simulink model "OvenSim"  (R2024a)
settings: Solver=FixedStepAuto  StartTime=0  StopTime=60  FixedStep=0.1  RelTol=1e-3
values from neighbouring files (symbols this model uses):
  A_innerwalls = 1.12    [ovenSimConfig.m]
  convection_loss_coefficient = 0.1    [ovenSimConfig.m]
  epsilon_food = 0.9    [ovenSimConfig.m]
  epsilon_innerWalls = 0.6    [ovenSimConfig.m]
  radiation_loss_coefficient = 0.24    [ovenSimConfig.m]
  sigma = 5.67e-8    (= 5.67e-08)    [ovenSimConfig.m]
undefined symbols (not defined in the file or in its folder): a, b
libraries: fl_lib x10, nesl_utility x8, CustomComponents_lib x1
settings Model: Creator=Jonas Zhou  LastModifiedBy=zhouziyao

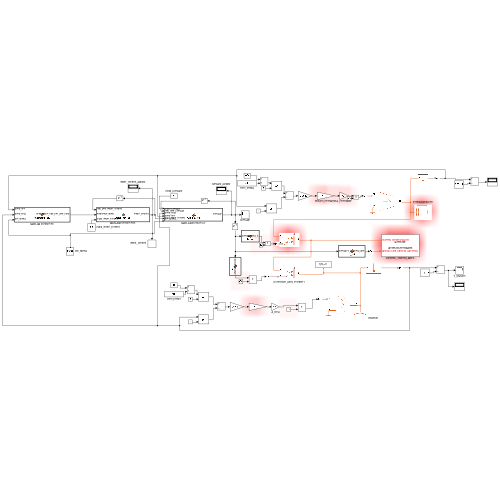
[thumbnail: Simulink's stored preview of the top-level diagram]
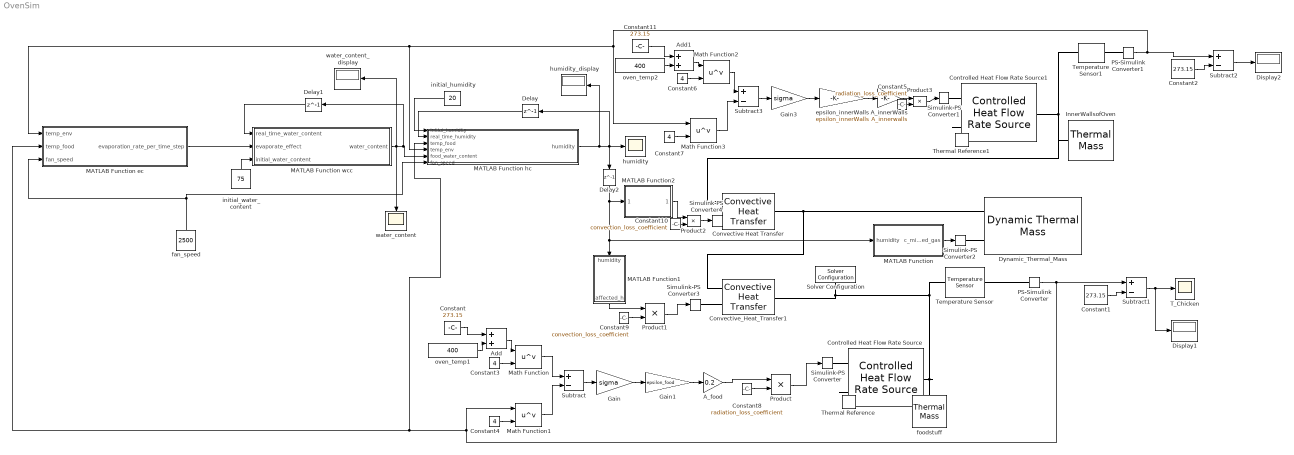
== system OvenSim ==
  A_food : Gain  Gain=0.2
  A_innerWalls : Gain  Gain=A_innerwalls
  Add : Sum
  Add1 : Sum
  Constant{,1..2,11} (4 alike) : Constant  Value=273.15
  Constant10 : Constant  Value=convection_loss_coefficient
  Constant{3..4,6..7} (4 alike) : Constant  Value=4
  Constant5 : Constant  Value=radiation_loss_coefficient
  Constant8 : Constant  Value=radiation_loss_coefficient
  Constant9 : Constant  Value=convection_loss_coefficient
  Controlled Heat Flow Rate Source : fl_lib/Thermal/Thermal Sources/Controlled Heat Flow Rate Source
  Controlled Heat Flow Rate Source1 : fl_lib/Thermal/Thermal Sources/Controlled Heat Flow Rate Source
  Convective Heat Transfer : fl_lib/Thermal/Thermal Elements/Convective Heat Transfer  thermal_type=foundation.enum.constant_variable.variable  area=A_gas m^2  heat_tr_coeff=h_innerwalls W/(K*m^2)  min_heat_tr_coeff=1e-3 W/(K*m^2)  T_specify=off  T_priority=None  T=a-b K  T_nominal_specify=off  T_nominal_value=1  T_nominal_unit=K  Q_specify=off  Q_priority=None  Q=0 W  Q_nominal_specify=off  Q_nominal_value=1  Q_nominal_unit=W
      settings: InternalSimscapePortConfiguration="{\"Bottom\":[],\"Left\":[{\"id\":\"A\",\"label\":\"A\",\"type\":\"foundation.thermal.thermal\"},{\"id\":\"var_heat_tr_coeff\",\"label\":\"K\",\"type\":\"input\"}],\"Right\":[{\"id\":\"B\",\"label\":\"B\",\"type\":\"foundation.thermal.thermal\"}],\"Top\":[]}"
  Convective_Heat_Transfer1 : fl_lib/Thermal/Thermal Elements/Convective Heat Transfer  thermal_type=foundation.enum.constant_variable.variable  area=0.2 m^2  heat_tr_coeff=20 W/(K*m^2)  min_heat_tr_coeff=1e-3 W/(K*m^2)  T_specify=off  T_priority=None  T=a-b K  T_nominal_specify=off  T_nominal_value=1  T_nominal_unit=K  Q_specify=off  Q_priority=None  Q=0 W  Q_nominal_specify=off  Q_nominal_value=1  Q_nominal_unit=W
      settings: InternalSimscapePortConfiguration="{\"Bottom\":[],\"Left\":[{\"id\":\"A\",\"label\":\"A\",\"type\":\"foundation.thermal.thermal\"},{\"id\":\"var_heat_tr_coeff\",\"label\":\"K\",\"type\":\"input\"}],\"Right\":[{\"id\":\"B\",\"label\":\"B\",\"type\":\"foundation.thermal.thermal\"}],\"Top\":[]}"
  Delay : Delay  DelayLength=1  InitialCondition=0
  Delay1 : Delay  DelayLength=1  InitialCondition=0
  Delay2 : Delay  DelayLength=1  InitialCondition=0
  Display1 : Display
  Display2 : Display
  Dynamic_Thermal_Mass : CustomComponents_lib/Dynamic Thermal Mass  mass=m_gas kg  T_specify=on  T_priority=None  T=400 degC  T_nominal_specify=off  T_nominal_value=1  T_nominal_unit=K  Q_specify=off  Q_priority=None  Q=0 W  Q_nominal_specify=off  Q_nominal_value=1  Q_nominal_unit=W
      settings: InternalSimscapePortConfiguration="{\"Bottom\":[],\"Left\":[{\"id\":\"M\",\"label\":\"Thermal conserving port\",\"type\":\"foundation.thermal.thermal\"},{\"id\":\"Cp\",\"label\":\"Specific heat capacity (dynamic)\",\"type\":\"input\"}],\"Right\":[],\"Top\":[]}"
  Gain : Gain  Gain=sigma
  Gain1 : Gain  Gain=epsilon_food
  Gain3 : Gain  Gain=sigma
  InnerWallsofOven : fl_lib/Thermal/Thermal Elements/Thermal Mass  mass_type=foundation.enum.constant_variable.constant  mass=m_innerwalls kg  sp_heat=c_innerwalls J/(K*kg)  mass_min=1e-6 kg  num_ports=foundation.enum.numPorts2.one  m_specify=off  m_priority=High  m=1 kg  m_nominal_specify=off  m_nominal_value=1  m_nominal_unit=kg  T_specify=on  T_priority=High  T=400 degC  T_nominal_specify=off  T_nominal_value=1  T_nominal_unit=K  Q_specify=off  Q_priority=None  Q=0 W  Q_nominal_specify=off  Q_nominal_value=1  Q_nominal_unit=W
  MATLAB Function : MATLAB Function  TreatAsAtomicUnit=on
  MATLAB Function ec : MATLAB Function  TreatAsAtomicUnit=on  SystemSampleTime=0.1
  MATLAB Function hc : MATLAB Function  TreatAsAtomicUnit=on
  MATLAB Function wcc : MATLAB Function  TreatAsAtomicUnit=on
  MATLAB Function1 : MATLAB Function  TreatAsAtomicUnit=on
  MATLAB Function2 : MATLAB Function  TreatAsAtomicUnit=on
  Math Function{,1..3} (4 alike) : Math  Operator=pow
  PS-Simulink Converter : nesl_utility/PS-Simulink Converter  PhysicalDomain=network_engine_domain  SubClassName=ps_output  LeftPortType=input  RightPortType=output  PseudoPeriodic=off  Frequencies=[]  VectorFormat=inherit  Unit=inherit  AffineConversion=off
  PS-Simulink Converter1 : nesl_utility/PS-Simulink Converter  PhysicalDomain=network_engine_domain  SubClassName=ps_output  LeftPortType=input  RightPortType=output  PseudoPeriodic=off  Frequencies=[]  VectorFormat=inherit  Unit=inherit  AffineConversion=off
  Product{,1..3} (4 alike) : Product
  Simulink-PS Converter{,1..4} (5 alike) : nesl_utility/Simulink-PS Converter  PhysicalDomain=network_engine_domain  SubClassName=ps_input  LeftPortType=input  RightPortType=output  PseudoPeriodic=off  Frequencies=[]  NoiseDistribution=none  NoiseParameters=[]  Unit=1  AffineConversion=off  FilteringAndDerivatives=provide  SimscapeFilterOrder=1  InputFilterTimeConstant=0.001  UdotUserProvided=0
  Solver Configuration : nesl_utility/Solver Configuration  PhysicalDomain=network_engine_domain  SubClassName=solver  LeftPortType=input  RightPortType=generic  Tones=[]  Harmonics=[]  SimulateNoise=off  Profile=off  UseLocalSampling=off  EnableSwitchedLinearOptims=on  FrequencyDomain=off  UseCCode=off  RelTol=0.001  AbsTol=0.001  MinStep=1e-09  ToWorkspace=off  RevertToSquareIcSolve=off  NumHomotopyIterations=100  PhasorMode=off  PhasorModeNumHarmonics=1  ConsistencySolver=NEWTON_XTOL_AFTER_FTOL  IndexReductionMethod=DerivativeReplacement  DoDC=off  ResidualTolerance=1e-09  ConsistencyTolSource=GLOBAL  ConsistencyAbsTol=0.001  ConsistencyRelTol=0.001  ConsistencyTolFactor=0.001  UseLocalSolver=off  LocalSolverChoice=NE_BACKWARD_EULER_ADVANCER  ResolveIndetEquations=on  FunctionEvalNumThread=1  LocalSolverSampleTime=0.001  DoFixedCost=off  MaxNonlinIter=3  MaxModeIter=2  ComputeImpulses=off  ImpulseIterations=2  LinearAlgebra=auto  LinearAlgebraNumThread=0  EquationFormulation=NE_TIME_EF  DelaysMemoryBudget=1024  AutomaticFiltering=on  FilteringTimeConstant=0.001  PartitionStorageMethod=AS_NEEDED  PartitionMemoryBudget=1024  PartitionMethod=ROBUST  MultibodyUseLocalSolver=off  MultibodyLocalSolverChoice=ODE1  MultibodyLocalSolverSampleTime=0.001
  Subtract{,1..3} (4 alike) : Sum  Inputs=+-
  T_Chicken : Scope
  Temperature Sensor : fl_lib/Thermal/Thermal Sensors/Temperature Sensor  temperature_measure=foundation.enum.MeasurementReference.absolute
      settings: InternalSimscapePortConfiguration="{\"Bottom\":[],\"Left\":[{\"id\":\"A\",\"label\":\"A\",\"type\":\"foundation.thermal.thermal\"}],\"Right\":[{\"id\":\"T\",\"label\":\"T\",\"type\":\"output\"}],\"Top\":[]}"
  Temperature Sensor1 : fl_lib/Thermal/Thermal Sensors/Temperature Sensor  temperature_measure=foundation.enum.MeasurementReference.absolute
      settings: InternalSimscapePortConfiguration="{\"Bottom\":[],\"Left\":[{\"id\":\"A\",\"label\":\"A\",\"type\":\"foundation.thermal.thermal\"}],\"Right\":[{\"id\":\"T\",\"label\":\"T\",\"type\":\"output\"}],\"Top\":[]}"
  Thermal Reference : fl_lib/Thermal/Thermal Elements/Thermal Reference
  Thermal Reference1 : fl_lib/Thermal/Thermal Elements/Thermal Reference
  epsilon_innerWalls : Gain  Gain=epsilon_innerWalls
  fan_speed : Constant  Value=2500
  foodstuff : fl_lib/Thermal/Thermal Elements/Thermal Mass  mass_type=foundation.enum.constant_variable.constant  mass=1.3 kg  sp_heat=3000 J/(K*kg)  mass_min=1e-6 kg  num_ports=foundation.enum.numPorts2.one  m_specify=off  m_priority=High  m=1 kg  m_nominal_specify=off  m_nominal_value=1  m_nominal_unit=kg  T_specify=on  T_priority=High  T=7 degC  T_nominal_specify=off  T_nominal_value=1  T_nominal_unit=K  Q_specify=off  Q_priority=None  Q=0 W  Q_nominal_specify=off  Q_nominal_value=1  Q_nominal_unit=W
  humidity : Scope
  humidity_display : Display
  initial_humidity : Constant  Value=20
  initial_water_content : Constant  Value=75
  oven_temp1 : Constant  Value=400
  oven_temp2 : Constant  Value=400
  water_content : Scope
  water_content_display : Display
  wires:
  PS-Simulink Converter1/1 -> Subtract2/1, MATLAB Function hc/4(temp_env), MATLAB Function ec/1(temp_env), Math Function3/1
  Gain3/1 -> epsilon_innerWalls/1
  Math Function3/1 -> Subtract3/2
  Constant7/1 -> Math Function3/2
  Subtract3/1 -> Gain3/1
  epsilon_innerWalls/1 -> A_innerWalls/1
  Math Function2/1 -> Subtract3/1
  Constant2/1 -> Subtract2/2
  Constant6/1 -> Math Function2/2
  Subtract2/1 -> Display2/1
  Constant4/1 -> Math Function1/2
  Math Function/1 -> Subtract/1
  Gain/1 -> Gain1/1
  Gain1/1 -> A_food/1
  Constant3/1 -> Math Function/2
  PS-Simulink Converter/1 -> Subtract1/1, MATLAB Function hc/3(temp_food), MATLAB Function ec/2(temp_food), Math Function1/1
  Subtract1/1 -> Display1/1, T_Chicken/1
  Math Function1/1 -> Subtract/2
  Constant1/1 -> Subtract1/2
  Subtract/1 -> Gain/1
  MATLAB Function ec/1(evaporation_rate_per_time_step) -> MATLAB Function wcc/2(evaporate_effect)
  MATLAB Function wcc/1(water_content) -> water_content_display/1, MATLAB Function hc/5(food_water_content), Delay1/1, water_content/1
  MATLAB Function hc/1(humidity) -> humidity_display/1, Delay2/1, humidity/1, Delay/1
  fan_speed/1 -> MATLAB Function hc/6(fan_speed), MATLAB Function ec/3(fan_speed)
  Delay/1 -> MATLAB Function hc/2(real_time_humidity)
  Delay1/1 -> MATLAB Function wcc/1(real_time_water_content)
  MATLAB Function/1(c_mixtured_gas) -> Simulink-PS Converter2/1
  Delay2/1 -> MATLAB Function/1(humidity), MATLAB Function1/1(humidity), MATLAB Function2/1(humidity)
  initial_water_content/1 -> MATLAB Function wcc/3(initial_water_content)
  Constant8/1 -> Product/2
  A_food/1 -> Product/1
  Constant9/1 -> Product1/2
  Product1/1 -> Simulink-PS Converter3/1
  MATLAB Function1/1(affected_h) -> Product1/1
  Constant10/1 -> Product2/2
  Product2/1 -> Simulink-PS Converter4/1
  MATLAB Function2/1(affected_h) -> Product2/1
  Product/1 -> Simulink-PS Converter/1
  A_innerWalls/1 -> Product3/1
  Constant5/1 -> Product3/2
  Product3/1 -> Simulink-PS Converter1/1
  Constant/1 -> Add/1
  oven_temp1/1 -> Add/2
  Add/1 -> Math Function/1
  Constant11/1 -> Add1/1
  oven_temp2/1 -> Add1/2
  Add1/1 -> Math Function2/1
  initial_humidity/1 -> MATLAB Function hc/1(initial_humidity)
  connections:
  Temperature Sensor1/LConn1 -- Convective Heat Transfer/LConn1 -- InnerWallsofOven/LConn1 -- Controlled Heat Flow Rate Source1/LConn1
  Controlled Heat Flow Rate Source1/RConn2 -- Thermal Reference1/LConn1
  Temperature Sensor1/RConn1 -- PS-Simulink Converter1/LConn1
  Convective_Heat_Transfer1/LConn1 -- Dynamic_Thermal_Mass/LConn1 -- Convective Heat Transfer/RConn1
  Solver Configuration/RConn1 -- Controlled Heat Flow Rate Source/LConn1 -- foodstuff/LConn1 -- Temperature Sensor/LConn1 -- Convective_Heat_Transfer1/RConn1
  Controlled Heat Flow Rate Source/RConn2 -- Thermal Reference/LConn1
  Temperature Sensor/RConn1 -- PS-Simulink Converter/LConn1
  Simulink-PS Converter2/RConn1 -- Dynamic_Thermal_Mass/LConn2
  Simulink-PS Converter3/RConn1 -- Convective_Heat_Transfer1/LConn2
  Simulink-PS Converter4/RConn1 -- Convective Heat Transfer/LConn2
  Simulink-PS Converter/RConn1 -- Controlled Heat Flow Rate Source/RConn1
  Simulink-PS Converter1/RConn1 -- Controlled Heat Flow Rate Source1/RConn1

== matlab function OvenSim/MATLAB Function ec ==
  data: temp_env input; temp_food input; fan_speed input; evaporation_rate_per_time_step output
function evaporation_rate_per_time_step = evaporate_cal(temp_env,temp_food,fan_speed)

% coefficient of temperature and fan speed 
k1=0.01*0.0035;
k2=0.00075*0.0035;

% adjustment for time step
k_step=0.1;

evaporation_rate_per_time_step=(k1*(temp_env-temp_food)+k2*fan_speed)*k_step;

end

== matlab function OvenSim/MATLAB Function hc ==
  settings: updateMethod=DISCRETE  sampleTime=0.1
  data: initial_humidity input; real_time_humidity input; temp_food input; humidity output; temp_env input; food_water_content input; fan_speed input
function humidity = humidity_cal(initial_humidity,real_time_humidity,temp_food,temp_env,food_water_content,fan_speed)

% coefficient of temperature,tuned according the humidity baseline
k1=0.0004;

% coefficient of fan speed,tuned according the humidity baseline
k2=0.000013;

% step coefficient
k_step=0.1;

persistent i;
if isempty(i)
    i=0;
end
if i==0
    
    humidity = initial_humidity+k1*(temp_env-temp_food)*food_water_content*0.01-k2*fan_speed;
    i=i+1;
else
    humidity = real_time_humidity + (k1*(temp_env-temp_food)*food_water_content*0.01-k2*fan_speed) *k_step;
end

if humidity > 100
    humidity = 100;
    elseif humidity < 0
        humidity = 0;
end

end

== matlab function OvenSim/MATLAB Function wcc ==
  settings: updateMethod=DISCRETE  sampleTime=0.1
  data: real_time_water_content input; water_content output; evaporate_effect input; initial_water_content input
function water_content = water_con_cal(real_time_water_content, evaporate_effect,initial_water_content)
    persistent i;
    if isempty(i)
        i = 0;
    end

    if i == 0
        % initial water content of chicken is 75%
        water_content = initial_water_content - evaporate_effect;
        i = i + 1;
    else
        water_content = real_time_water_content - evaporate_effect;
    end

    if water_content < 0
        water_content = 0.1;
    end
end

== matlab function OvenSim/MATLAB Function ==
  data: humidity input; c_mixtured_gas output
function c_mixtured_gas = c_cal(humidity)

c_mixtured_gas = (1.005+humidity*0.01*(1.84-1.005))*1000;

== matlab function OvenSim/MATLAB Function1 ==
  data: humidity input; affected_h output
function affected_h = h_cal(humidity)

affected_h = (0.026+humidity*0.01*(0.018-0.026))*199.18;

== matlab function OvenSim/MATLAB Function2 ==
  data: humidity input; affected_h output
function affected_h = h_cal(humidity)

affected_h = (0.026+humidity*0.01*(0.018-0.026))*199.18;
